simulink model "SGBMDisparityCopy"  (R2021a)
settings: Solver=FixedStepDiscrete  StartTime=0.0  StopTime=simT  FixedStep=1  RelTol=1e-3
PreLoadFcn:
  | DL128 = Simulink.Variant('disparityLevels==128');
  | 
  | DLnot128 = Simulink.Variant('disparityLevels ~= 128');
  | 
  | disparityLevels = 64;
  | 
  | imgRowSize = 480;
  | 
  | imgColSize = 640;
  | 
  | P2 = 200; % Smoothness Penalty Large
  | P1 = 15;  % Smoothness Penalty Small
  | 
  | disparityFactor = 16;
  | 
  | uniquenessRatio = 5;
  | 
  | p = imgColSize - 1;
  | q = imgRowSize * imgColSize -1;
  | r = imgColSize - disparityLevels -1;
  | s = (imgRowSize*(imgColSize-disparityLevels))-1;
  | 
  | simT = 800*525
  | 
  | dtGain = 4;
InitFcn:
  | DL128 = Simulink.Variant('disparityLevels==128');
  | 
  | DLnot128 = Simulink.Variant('disparityLevels ~= 128');
  | 
  | img = imread(get_param('SGBMDisparity/stereoImage','FileName'));
  | 
  | [imgRowSize, imgColSize,chn] = size(img);
  | 
  | P2 = 200; % Smoothness Penalty Large
  | P1 = 15;  % Smoothness Penalty Small
  | 
  | disparityFactor = 16;
  | 
  | uniquenessRatio = str2num(get_param('SGBMDisparity/SGBMHDLAlgorithm/SGBMHDLAlgorithmWorker','UT'));
  | 
  | disparityLevels = str2num(get_param('SGBMDisparity/SGBMHDLAlgorithm/SGBMHDLAlgorithmWorker','DL'));
  | 
  | p = imgColSize - 1;
  | q = imgRowSize * imgColSize -1;
  | r = imgColSize - disparityLevels -1;
  | s = (imgRowSize*(imgColSize-disparityLevels))-1;
  | 
  | if imgRowSize == 720 && imgColSize == 1280
  | simT = 1650*750;
  | elseif imgRowSize == 540 && imgColSize == 960
  | simT = 1050*600;
  | elseif imgRowSize == 480 && imgColSize == 640
  | simT = 800*525;
  | end
  | 
  | if imgRowSize == 720 && imgColSize == 1280
  | dtGain = 2;
  | elseif imgRowSize == 540 && imgColSize == 960
  | dtGain = 2.6;
  | elseif imgRowSize == 480 && imgColSize == 640
  | dtGain = 4;
  | end
undefined symbols (not defined in the file or in its folder): gray
libraries: simulink x331, hdlsllib x113, visionhdlutilities x9, visionhdlio x2, visionsources x1
(part 4 of 6)

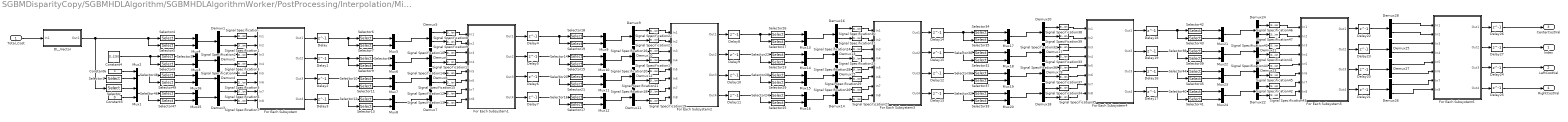
== system SGBMDisparityCopy/SGBMHDLAlgorithm/SGBMHDLAlgorithmWorker/PostProcessing/Interpolation/Minimum_Cost_Index ==
  Total_Cost : Inport
  Constant4 : Constant  Value=[1:128]  OutDataTypeStr=uint8  SampleTime=-1
  Constant5 : Constant  Value=0  OutDataTypeStr=fixdt(1,13,0)  SampleTime=-1
  Constant6 : Constant  Value=0  OutDataTypeStr=fixdt(1,13,0)  SampleTime=-1
  DL_Vector : Subsystem  Variant=on
  Delay{,1..27} (28 alike) : Delay  DelayLength=1
  Demux{1..28} (28 alike) : Demux  Outputs=2
  For Each Subsystem : Subsystem  TreatAsAtomicUnit=on
  For Each Subsystem1 : Subsystem  TreatAsAtomicUnit=on
  For Each Subsystem2 : Subsystem  TreatAsAtomicUnit=on
  For Each Subsystem3 : Subsystem  TreatAsAtomicUnit=on
  For Each Subsystem4 : Subsystem  TreatAsAtomicUnit=on
  For Each Subsystem5 : Subsystem  TreatAsAtomicUnit=on
  For Each Subsystem6 : Subsystem  TreatAsAtomicUnit=on
  Mux{1..26} (26 alike) : Mux  Inputs=2
  Selector : Selector  InputPortWidth=128  IndexOptions=Index vector (dialog)  Indices=[2:128]  OutputSizes=1
  Selector1 : Selector  InputPortWidth=128  IndexOptions=Index vector (dialog)  Indices=[1:127]  OutputSizes=1
  Selector{6,8,10,12} (4 alike) : Selector  InputPortWidth=64  IndexOptions=Index vector (dialog)  Indices=[1:2:64]  OutputSizes=1
  Selector{7,9,11,13} (4 alike) : Selector  InputPortWidth=64  IndexOptions=Index vector (dialog)  Indices=[2:2:64]  OutputSizes=1
  Selector{14,16,18,20} (4 alike) : Selector  InputPortWidth=32  IndexOptions=Index vector (dialog)  Indices=[1:2:32]  OutputSizes=1
  Selector{15,17,19,21} (4 alike) : Selector  InputPortWidth=32  IndexOptions=Index vector (dialog)  Indices=[2:2:32]  OutputSizes=1
  Selector{2,4,46,48} (4 alike) : Selector  InputPortWidth=128  IndexOptions=Index vector (dialog)  Indices=[1:2:128]  OutputSizes=1
  Selector{22,24,26,28} (4 alike) : Selector  InputPortWidth=16  IndexOptions=Index vector (dialog)  Indices=[1:2:16]  OutputSizes=1
  Selector{23,25,27,29} (4 alike) : Selector  InputPortWidth=16  IndexOptions=Index vector (dialog)  Indices=[2:2:16]  OutputSizes=1
  Selector{3,5,47,49} (4 alike) : Selector  InputPortWidth=128  IndexOptions=Index vector (dialog)  Indices=[2:2:128]  OutputSizes=1
  Selector{30,32,34,36} (4 alike) : Selector  InputPortWidth=8  IndexOptions=Index vector (dialog)  Indices=[1:2:8]  OutputSizes=1
  Selector{31,33,35,37} (4 alike) : Selector  InputPortWidth=8  IndexOptions=Index vector (dialog)  Indices=[2:2:8]  OutputSizes=1
  Selector{38,40,42,44} (4 alike) : Selector  InputPortWidth=4  IndexOptions=Index vector (dialog)  Indices=[1:2:4]  OutputSizes=1
  Selector{39,41,43,45} (4 alike) : Selector  InputPortWidth=4  IndexOptions=Index vector (dialog)  Indices=[2:2:4]  OutputSizes=1
  Signal Specification{,1..7} (8 alike) : SignalSpecification  Dimensions=64
  Signal Specification{8..15} (8 alike) : SignalSpecification  Dimensions=32
  Signal Specification{16..23} (8 alike) : SignalSpecification  Dimensions=16
  Signal Specification{24..31} (8 alike) : SignalSpecification  Dimensions=8
  Signal Specification{32..39} (8 alike) : SignalSpecification  Dimensions=4
  Signal Specification{40..47} (8 alike) : SignalSpecification  Dimensions=2
  Index : Outport  VectorParamsAs1DForOutWhenUnconnected=off
  LeftCostVal : Outport  Port=2  VectorParamsAs1DForOutWhenUnconnected=off
  CenterCostVal : Outport  Port=3  VectorParamsAs1DForOutWhenUnconnected=off
  RightCostVal : Outport  Port=4  VectorParamsAs1DForOutWhenUnconnected=off
  wires:
  Demux1/1 -> Signal Specification/1
  Demux1/2 -> Signal Specification1/1
  Demux4/1 -> Signal Specification4/1
  Selector1/1 -> Mux2/2
  Demux2/2 -> Signal Specification3/1
  Demux3/1 -> Signal Specification6/1
  Selector/1 -> Mux1/1
  Demux3/2 -> Signal Specification7/1
  Constant6/1 -> Mux2/1
  Constant5/1 -> Mux1/2
  Demux4/2 -> Signal Specification5/1
  Demux2/1 -> Signal Specification2/1
  Signal Specification/1 -> For Each Subsystem/1(In1)
  Signal Specification1/1 -> For Each Subsystem/2(In2)
  Signal Specification2/1 -> For Each Subsystem/3(In3)
  Signal Specification3/1 -> For Each Subsystem/4(In4)
  Signal Specification4/1 -> For Each Subsystem/5(In5)
  Signal Specification7/1 -> For Each Subsystem/8(In8)
  Signal Specification6/1 -> For Each Subsystem/7(In7)
  Signal Specification5/1 -> For Each Subsystem/6(In6)
  Demux5/1 -> Signal Specification8/1
  For Each Subsystem/1(Out1) -> Delay/1
  Demux6/2 -> Signal Specification11/1
  For Each Subsystem/2(Out2) -> Delay1/1
  Demux5/2 -> Signal Specification9/1
  Demux6/1 -> Signal Specification10/1
  For Each Subsystem/3(Out3) -> Delay2/1
  Demux7/2 -> Signal Specification13/1
  For Each Subsystem/4(Out4) -> Delay3/1
  Demux8/1 -> Signal Specification14/1
  Demux8/2 -> Signal Specification15/1
  Demux7/1 -> Signal Specification12/1
  Signal Specification8/1 -> For Each Subsystem1/1(In1)
  Signal Specification9/1 -> For Each Subsystem1/2(In2)
  Signal Specification10/1 -> For Each Subsystem1/3(In3)
  Signal Specification11/1 -> For Each Subsystem1/4(In4)
  Signal Specification14/1 -> For Each Subsystem1/5(In5)
  Signal Specification15/1 -> For Each Subsystem1/6(In6)
  Signal Specification12/1 -> For Each Subsystem1/7(In7)
  Signal Specification13/1 -> For Each Subsystem1/8(In8)
  For Each Subsystem1/2(Out2) -> Delay5/1
  Signal Specification19/1 -> For Each Subsystem2/8(In8)
  Demux11/2 -> Signal Specification19/1
  Signal Specification18/1 -> For Each Subsystem2/7(In7)
  Signal Specification22/1 -> For Each Subsystem2/1(In1)
  Signal Specification16/1 -> For Each Subsystem2/3(In3)
  For Each Subsystem1/4(Out4) -> Delay7/1
  Signal Specification23/1 -> For Each Subsystem2/2(In2)
  Signal Specification17/1 -> For Each Subsystem2/4(In4)
  Demux10/1 -> Signal Specification16/1
  Demux9/2 -> Signal Specification23/1
  Demux12/1 -> Signal Specification20/1
  Signal Specification20/1 -> For Each Subsystem2/5(In5)
  For Each Subsystem1/1(Out1) -> Delay4/1
  Demux10/2 -> Signal Specification17/1
  Signal Specification21/1 -> For Each Subsystem2/6(In6)
  Demux11/1 -> Signal Specification18/1
  Demux9/1 -> Signal Specification22/1
  For Each Subsystem1/3(Out3) -> Delay6/1
  Demux12/2 -> Signal Specification21/1
  For Each Subsystem2/1(Out1) -> Delay8/1
  Demux14/1 -> Signal Specification26/1
  Demux16/1 -> Signal Specification30/1
  Demux13/2 -> Signal Specification25/1
  Demux15/2 -> Signal Specification29/1
  Demux15/1 -> Signal Specification28/1
  Demux13/1 -> Signal Specification24/1
  Demux16/2 -> Signal Specification31/1
  Demux14/2 -> Signal Specification27/1
  Signal Specification28/1 -> For Each Subsystem3/5(In5)
  Signal Specification26/1 -> For Each Subsystem3/7(In7)
  Signal Specification24/1 -> For Each Subsystem3/3(In3)
  Signal Specification29/1 -> For Each Subsystem3/6(In6)
  For Each Subsystem2/4(Out4) -> Delay11/1
  Signal Specification25/1 -> For Each Subsystem3/4(In4)
  Signal Specification31/1 -> For Each Subsystem3/2(In2)
  For Each Subsystem2/2(Out2) -> Delay9/1
  For Each Subsystem2/3(Out3) -> Delay10/1
  Signal Specification27/1 -> For Each Subsystem3/8(In8)
  Signal Specification30/1 -> For Each Subsystem3/1(In1)
  For Each Subsystem3/1(Out1) -> Delay14/1
  Demux18/1 -> Signal Specification34/1
  Demux20/1 -> Signal Specification38/1
  Demux17/2 -> Signal Specification33/1
  Demux19/2 -> Signal Specification37/1
  Demux19/1 -> Signal Specification36/1
  Demux17/1 -> Signal Specification32/1
  Demux20/2 -> Signal Specification39/1
  Demux18/2 -> Signal Specification35/1
  Signal Specification36/1 -> For Each Subsystem4/5(In5)
  Signal Specification34/1 -> For Each Subsystem4/7(In7)
  Signal Specification32/1 -> For Each Subsystem4/3(In3)
  Signal Specification37/1 -> For Each Subsystem4/6(In6)
  For Each Subsystem3/4(Out4) -> Delay13/1
  Signal Specification33/1 -> For Each Subsystem4/4(In4)
  Signal Specification39/1 -> For Each Subsystem4/2(In2)
  For Each Subsystem3/2(Out2) -> Delay15/1
  For Each Subsystem3/3(Out3) -> Delay12/1
  Signal Specification35/1 -> For Each Subsystem4/8(In8)
  Signal Specification38/1 -> For Each Subsystem4/1(In1)
  For Each Subsystem4/1(Out1) -> Delay18/1
  For Each Subsystem4/4(Out4) -> Delay17/1
  For Each Subsystem4/2(Out2) -> Delay19/1
  For Each Subsystem4/3(Out3) -> Delay16/1
  Constant4/1 -> Selector3/1, Selector2/1
  Selector2/1 -> Mux3/1
  Selector3/1 -> Mux3/2
  Mux3/1 -> Demux2/1
  Selector4/1 -> Mux4/1
  Selector5/1 -> Mux4/2
  Mux4/1 -> Demux1/1
  Demux24/1 -> Signal Specification46/1
  Demux24/2 -> Signal Specification47/1
  Demux22/2 -> Signal Specification43/1
  Demux21/2 -> Signal Specification41/1
  Demux23/2 -> Signal Specification45/1
  Demux23/1 -> Signal Specification44/1
  Demux21/1 -> Signal Specification40/1
  Demux22/1 -> Signal Specification42/1
  For Each Subsystem5/2(Out2) -> Delay23/1
  For Each Subsystem5/3(Out3) -> Delay20/1
  For Each Subsystem5/4(Out4) -> Delay21/1
  For Each Subsystem5/1(Out1) -> Delay22/1
  Selector6/1 -> Mux5/1
  Selector7/1 -> Mux5/2
  Delay/1 -> Selector7/1, Selector6/1
  Mux5/1 -> Demux5/1
  Selector8/1 -> Mux6/1
  Selector9/1 -> Mux6/2
  Delay1/1 -> Selector8/1, Selector9/1
  Mux6/1 -> Demux6/1
  Mux7/1 -> Demux8/1
  Selector11/1 -> Mux7/2
  Delay2/1 -> Selector11/1, Selector10/1
  Selector10/1 -> Mux7/1
  Mux8/1 -> Demux7/1
  Selector13/1 -> Mux8/2
  Delay3/1 -> Selector12/1, Selector13/1
  Selector12/1 -> Mux8/1
  Selector20/1 -> Mux11/1
  Selector21/1 -> Mux11/2
  Delay5/1 -> Selector15/1, Selector14/1
  Mux10/1 -> Demux10/1
  Delay6/1 -> Selector20/1, Selector21/1
  Selector17/1 -> Mux12/2
  Mux11/1 -> Demux12/1
  Selector16/1 -> Mux12/1
  Selector15/1 -> Mux10/2
  Mux9/1 -> Demux9/1
  Selector19/1 -> Mux9/2
  Delay4/1 -> Selector19/1, Selector18/1
  Selector18/1 -> Mux9/1
  Selector14/1 -> Mux10/1
  Mux12/1 -> Demux11/1
  Delay7/1 -> Selector17/1, Selector16/1
  Selector28/1 -> Mux15/1
  Selector29/1 -> Mux15/2
  Delay9/1 -> Selector23/1, Selector22/1
  Mux14/1 -> Demux13/1
  Delay10/1 -> Selector29/1, Selector28/1
  Selector25/1 -> Mux16/2
  Mux15/1 -> Demux15/1
  Selector24/1 -> Mux16/1
  Selector23/1 -> Mux14/2
  Mux13/1 -> Demux16/1
  Selector27/1 -> Mux13/2
  Delay8/1 -> Selector27/1, Selector26/1
  Selector26/1 -> Mux13/1
  Selector22/1 -> Mux14/1
  Mux16/1 -> Demux14/1
  Delay11/1 -> Selector25/1, Selector24/1
  Selector36/1 -> Mux19/1
  Selector37/1 -> Mux19/2
  Delay15/1 -> Selector31/1, Selector30/1
  Mux18/1 -> Demux17/1
  Delay12/1 -> Selector37/1, Selector36/1
  Selector33/1 -> Mux20/2
  Mux19/1 -> Demux19/1
  Selector32/1 -> Mux20/1
  Selector31/1 -> Mux18/2
  Mux17/1 -> Demux20/1
  Selector35/1 -> Mux17/2
  Delay14/1 -> Selector35/1, Selector34/1
  Selector34/1 -> Mux17/1
  Selector30/1 -> Mux18/1
  Mux20/1 -> Demux18/1
  Delay13/1 -> Selector33/1, Selector32/1
  Selector44/1 -> Mux23/1
  Selector45/1 -> Mux23/2
  Delay19/1 -> Selector38/1, Selector39/1
  Mux22/1 -> Demux21/1
  Delay16/1 -> Selector45/1, Selector44/1
  Selector41/1 -> Mux24/2
  Mux23/1 -> Demux23/1
  Selector40/1 -> Mux24/1
  Selector39/1 -> Mux22/2
  Mux21/1 -> Demux24/1
  Selector43/1 -> Mux21/2
  Delay18/1 -> Selector43/1, Selector42/1
  Selector42/1 -> Mux21/1
  Selector38/1 -> Mux22/1
  Mux24/1 -> Demux22/1
  Delay17/1 -> Selector41/1, Selector40/1
  Mux2/1 -> Selector49/1, Selector48/1
  Mux25/1 -> Demux3/1
  Selector47/1 -> Mux25/2
  Selector48/1 -> Mux26/1
  Mux1/1 -> Selector47/1, Selector46/1
  Selector49/1 -> Mux26/2
  Mux26/1 -> Demux4/1
  Selector46/1 -> Mux25/1
  DL_Vector/1(Out1) -> Selector1/1, Selector/1, Selector5/1, Selector4/1
  Signal Specification42/1 -> For Each Subsystem5/7(In7)
  Signal Specification41/1 -> For Each Subsystem5/4(In4)
  Signal Specification40/1 -> For Each Subsystem5/3(In3)
  Signal Specification45/1 -> For Each Subsystem5/6(In6)
  Signal Specification46/1 -> For Each Subsystem5/1(In1)
  Signal Specification43/1 -> For Each Subsystem5/8(In8)
  Signal Specification44/1 -> For Each Subsystem5/5(In5)
  Signal Specification47/1 -> For Each Subsystem5/2(In2)
  For Each Subsystem6/2(Out2) -> Delay27/1
  For Each Subsystem6/3(Out3) -> Delay24/1
  Demux26/2 -> For Each Subsystem6/8(In8)
  Demux28/1 -> For Each Subsystem6/1(In1)
  Demux27/2 -> For Each Subsystem6/6(In6)
  Demux25/2 -> For Each Subsystem6/4(In4)
  For Each Subsystem6/4(Out4) -> Delay25/1
  Delay21/1 -> Demux26/1
  Delay20/1 -> Demux27/1
  Demux28/2 -> For Each Subsystem6/2(In2)
  For Each Subsystem6/1(Out1) -> Delay26/1
  Demux27/1 -> For Each Subsystem6/5(In5)
  Delay23/1 -> Demux25/1
  Demux25/1 -> For Each Subsystem6/3(In3)
  Demux26/1 -> For Each Subsystem6/7(In7)
  Delay22/1 -> Demux28/1
  Delay26/1 -> CenterCostVal/1
  Delay27/1 -> Index/1
  Delay24/1 -> LeftCostVal/1
  Delay25/1 -> RightCostVal/1
  Total_Cost/1 -> DL_Vector/1(In1)

== system SGBMDisparityCopy/SGBMHDLAlgorithm/SGBMHDLAlgorithmWorker/PostProcessing/UniquenessFcn/For Each Subsystem ==
  total_cost : Inport  Partition=on  PartitionDimension=1  PartitionWidth=1  PartitionOffset=0
  total_cost1 : Inport  Port=2
  min_index_val : Inport  Port=3
  Delay : Delay  DelayLength=1
  For Each : ForEach  DisableCoverage=on
  Product : Product  RndMeth=Simplest
  Relational Operator1 : RelationalOperator  Operator=<  OutDataTypeStr=boolean  RndMeth=Nearest
  Out1 : Outport  ConcatenationDimension=1  VectorParamsAs1DForOutWhenUnconnected=off
  wires:
  total_cost/1 -> Product/1
  total_cost1/1 -> Product/2
  Product/1 -> Delay/1
  Delay/1 -> Relational Operator1/1
  min_index_val/1 -> Relational Operator1/2
  Relational Operator1/1 -> Out1/1

== system SGBMDisparityCopy/SGBMHDLAlgorithm/SGBMHDLAlgorithmWorker/PostProcessing/UniquenessFcn/For Each Subsystem1 ==
  min_Index : Inport
  Index : Inport  Port=2  Partition=on  PartitionDimension=1  PartitionWidth=1  PartitionOffset=0
  Abs1 : Abs  RndMeth=Simplest  SaturateOnIntegerOverflow=on
  Add2 : Sum  Inputs=+-
  Constant63 : Constant  OutDataTypeStr=uint8  SampleTime=-1
  Delay133 : Delay  DelayLength=1
  Delay37 : Delay  DelayLength=1
  For Each : ForEach  DisableCoverage=on
  Relational Operator2 : RelationalOperator  Operator=>  OutDataTypeStr=boolean  RndMeth=Nearest
  Out1 : Outport  ConcatenationDimension=1  VectorParamsAs1DForOutWhenUnconnected=off
  wires:
  Add2/1 -> Delay133/1
  Constant63/1 -> Relational Operator2/2
  Abs1/1 -> Delay37/1
  Delay37/1 -> Relational Operator2/1
  Delay133/1 -> Abs1/1
  min_Index/1 -> Add2/1
  Index/1 -> Add2/2
  Relational Operator2/1 -> Out1/1

== system SGBMDisparityCopy/SGBMHDLAlgorithm/SGBMHDLAlgorithmWorker/DirectionalCost/LeftToRight/lrSubsystem/For Each Subsystem ==
  In1 : Inport  Partition=on  PartitionDimension=1  PartitionWidth=1  PartitionOffset=0
  Constant2 : Constant  Value=0  OutDataTypeStr=boolean  SampleTime=-1
  For Each : ForEach  DisableCoverage=on
  Terminator : Terminator
  Out1 : Outport  ConcatenationDimension=1  VectorParamsAs1DForOutWhenUnconnected=off
  wires:
  Constant2/1 -> Out1/1
  In1/1 -> Terminator/1

== system SGBMDisparityCopy/SGBMHDLAlgorithm/SGBMHDLAlgorithmWorker/DirectionalCost/LeftToRight/lrSubsystem/d+1 ==
  prevCost_d : Inport
  Constant : Constant  Value=255  OutDataTypeStr=fixdt(1,10,0)  SampleTime=-1
  Selector : Selector  InputPortWidth=disparityLevels  IndexOptions=Index vector (dialog)  Indices=[2:disparityLevels]  OutputSizes=1
  Vector Concatenate : Concatenate
  prevCost_d+1 : Outport  VectorParamsAs1DForOutWhenUnconnected=off
  wires:
  prevCost_d/1 -> Selector/1
  Vector Concatenate/1 -> prevCost_d+1/1
  Selector/1 -> Vector Concatenate/1
  Constant/1 -> Vector Concatenate/2

== system SGBMDisparityCopy/SGBMHDLAlgorithm/SGBMHDLAlgorithmWorker/DirectionalCost/LeftToRight/lrSubsystem/d-1 ==
  prevCost_d : Inport
  Constant : Constant  Value=255  OutDataTypeStr=fixdt(1,10,0)  SampleTime=-1
  Selector : Selector  InputPortWidth=disparityLevels  IndexOptions=Index vector (dialog)  Indices=[1:disparityLevels-1]  OutputSizes=1
  Vector Concatenate : Concatenate
  prevCost_d-1 : Outport  VectorParamsAs1DForOutWhenUnconnected=off
  wires:
  prevCost_d/1 -> Selector/1
  Vector Concatenate/1 -> prevCost_d-1/1
  Selector/1 -> Vector Concatenate/2
  Constant/1 -> Vector Concatenate/1

== system SGBMDisparityCopy/SGBMHDLAlgorithm/SGBMHDLAlgorithmWorker/DirectionalCost/LeftToRight/lrSubsystem/minCostPath ==
  matchingCost : Inport  Partition=on  PartitionDimension=1  PartitionWidth=1  PartitionOffset=0
  prevCost_d : Inport  Port=2  Partition=on  PartitionDimension=1  PartitionWidth=1  PartitionOffset=0
  prevCost_d-1 : Inport  Port=3  Partition=on  PartitionDimension=1  PartitionWidth=1  PartitionOffset=0
  prevCost_d+1 : Inport  Port=4  Partition=on  PartitionDimension=1  PartitionWidth=1  PartitionOffset=0
  minPrevCost : Inport  Port=5
  Constant : Constant  Value=P1  OutDataTypeStr=fixdt(0,5,0)  SampleTime=-1
  Constant1 : Constant  Value=P2  OutDataTypeStr=uint8  SampleTime=-1
  For Each : ForEach  DisableCoverage=on
  Min : MinMax  Inputs=4
  Sum : Sum  Inputs=|++  OutDataTypeStr=fixdt(0,13,0)  SaturateOnIntegerOverflow=on
  Sum1 : Sum  Inputs=++|  OutDataTypeStr=fixdt(0,13,0)  SaturateOnIntegerOverflow=on
  Sum2 : Sum  Inputs=++|  OutDataTypeStr=int16  SaturateOnIntegerOverflow=on
  Sum3 : Sum  OutDataTypeStr=fixdt(1,17,0)  SaturateOnIntegerOverflow=on
  Sum4 : Sum  Inputs=+-  OutDataTypeStr=fixdt(1,10,0)  SaturateOnIntegerOverflow=on
  currCost : Outport  ConcatenationDimension=1  VectorParamsAs1DForOutWhenUnconnected=off
  wires:
  Sum1/1 -> Min/3
  Sum2/1 -> Min/4
  minPrevCost/1 -> Sum4/2, Sum2/2
  Sum/1 -> Min/2
  Constant1/1 -> Sum2/1
  prevCost_d/1 -> Min/1
  prevCost_d-1/1 -> Sum/1
  Min/1 -> Sum3/2
  prevCost_d+1/1 -> Sum1/2
  Constant/1 -> Sum1/1, Sum/2
  matchingCost/1 -> Sum3/1
  Sum3/1 -> Sum4/1
  Sum4/1 -> currCost/1

== system SGBMDisparityCopy/SGBMHDLAlgorithm/SGBMHDLAlgorithmWorker/DirectionalCost/RightToLeft/rlSubsystem/For Each Subsystem ==
  In1 : Inport  Partition=on  PartitionDimension=1  PartitionWidth=1  PartitionOffset=0
  Constant2 : Constant  Value=0  OutDataTypeStr=boolean  SampleTime=-1
  For Each : ForEach  DisableCoverage=on
  Terminator : Terminator
  Out1 : Outport  ConcatenationDimension=1  VectorParamsAs1DForOutWhenUnconnected=off
  wires:
  Constant2/1 -> Out1/1
  In1/1 -> Terminator/1

== system SGBMDisparityCopy/SGBMHDLAlgorithm/SGBMHDLAlgorithmWorker/DirectionalCost/RightToLeft/rlSubsystem/d+1 ==
  prev_cost_d : Inport
  Constant : Constant  Value=255  OutDataTypeStr=fixdt(1,10,0)  SampleTime=-1
  Selector : Selector  InputPortWidth=disparityLevels  IndexOptions=Index vector (dialog)  Indices=[2:disparityLevels]  OutputSizes=1
  Vector Concatenate : Concatenate
  prev_cost_d+1 : Outport  VectorParamsAs1DForOutWhenUnconnected=off
  wires:
  prev_cost_d/1 -> Selector/1
  Vector Concatenate/1 -> prev_cost_d+1/1
  Selector/1 -> Vector Concatenate/1
  Constant/1 -> Vector Concatenate/2

== system SGBMDisparityCopy/SGBMHDLAlgorithm/SGBMHDLAlgorithmWorker/DirectionalCost/RightToLeft/rlSubsystem/d-1 ==
  prev_cost_d : Inport
  Constant : Constant  Value=255  OutDataTypeStr=fixdt(1,10,0)  SampleTime=-1
  Selector : Selector  InputPortWidth=disparityLevels  IndexOptions=Index vector (dialog)  Indices=[1:disparityLevels-1]  OutputSizes=1
  Vector Concatenate : Concatenate
  prev_cost_d-1 : Outport  VectorParamsAs1DForOutWhenUnconnected=off
  wires:
  prev_cost_d/1 -> Selector/1
  Vector Concatenate/1 -> prev_cost_d-1/1
  Selector/1 -> Vector Concatenate/2
  Constant/1 -> Vector Concatenate/1

== system SGBMDisparityCopy/SGBMHDLAlgorithm/SGBMHDLAlgorithmWorker/DirectionalCost/RightToLeft/rlSubsystem/minCostPath ==
  Matching_Cost : Inport  Partition=on  PartitionDimension=1  PartitionWidth=1  PartitionOffset=0
  prev_cost_d : Inport  Port=2  Partition=on  PartitionDimension=1  PartitionWidth=1  PartitionOffset=0
  prev_cost_d-1 : Inport  Port=3  Partition=on  PartitionDimension=1  PartitionWidth=1  PartitionOffset=0
  prev_cost_d+1 : Inport  Port=4  Partition=on  PartitionDimension=1  PartitionWidth=1  PartitionOffset=0
  min_prev_cost : Inport  Port=5
  Constant : Constant  Value=P1  OutDataTypeStr=fixdt(0,5,0)  SampleTime=-1
  Constant1 : Constant  Value=P2  OutDataTypeStr=uint8  SampleTime=-1
  For Each : ForEach  DisableCoverage=on
  Min : MinMax  Inputs=4
  Sum : Sum  Inputs=|++  OutDataTypeStr=fixdt(0,13,0)  SaturateOnIntegerOverflow=on
  Sum1 : Sum  Inputs=++|  OutDataTypeStr=fixdt(0,13,0)  SaturateOnIntegerOverflow=on
  Sum2 : Sum  Inputs=++|  OutDataTypeStr=int16  SaturateOnIntegerOverflow=on
  Sum3 : Sum  OutDataTypeStr=fixdt(1,17,0)  SaturateOnIntegerOverflow=on
  Sum4 : Sum  Inputs=+-  OutDataTypeStr=fixdt(1,10,0)  SaturateOnIntegerOverflow=on
  curr_cost : Outport  ConcatenationDimension=1  VectorParamsAs1DForOutWhenUnconnected=off
  wires:
  Sum1/1 -> Min/3
  Sum2/1 -> Min/4
  Sum3/1 -> Sum4/1
  min_prev_cost/1 -> Sum4/2, Sum2/2
  Sum/1 -> Min/2
  Constant1/1 -> Sum2/1
  prev_cost_d/1 -> Min/1
  prev_cost_d-1/1 -> Sum/1
  Min/1 -> Sum3/2
  prev_cost_d+1/1 -> Sum1/2
  Constant/1 -> Sum1/1, Sum/2
  Matching_Cost/1 -> Sum3/1
  Sum4/1 -> curr_cost/1

== system SGBMDisparityCopy/SGBMHDLAlgorithm/SGBMHDLAlgorithmWorker/DirectionalCost/TopLeftToBottomRight/tlbrSubsystem/For Each Subsystem ==
  In1 : Inport  Partition=on  PartitionDimension=1  PartitionWidth=1  PartitionOffset=0
  Constant2 : Constant  Value=0  OutDataTypeStr=boolean  SampleTime=-1
  For Each : ForEach  DisableCoverage=on
  Terminator : Terminator
  Out1 : Outport  ConcatenationDimension=1  VectorParamsAs1DForOutWhenUnconnected=off
  wires:
  Constant2/1 -> Out1/1
  In1/1 -> Terminator/1

== system SGBMDisparityCopy/SGBMHDLAlgorithm/SGBMHDLAlgorithmWorker/DirectionalCost/TopLeftToBottomRight/tlbrSubsystem/d+2 ==
  prev_cost_d : Inport
  Constant : Constant  Value=255  OutDataTypeStr=fixdt(1,10,0)  SampleTime=-1
  Selector : Selector  InputPortWidth=disparityLevels  IndexOptions=Index vector (dialog)  Indices=[2:disparityLevels]  OutputSizes=1
  Vector Concatenate : Concatenate
  prev_cost_d+1 : Outport  VectorParamsAs1DForOutWhenUnconnected=off
  wires:
  prev_cost_d/1 -> Selector/1
  Vector Concatenate/1 -> prev_cost_d+1/1
  Selector/1 -> Vector Concatenate/1
  Constant/1 -> Vector Concatenate/2

== system SGBMDisparityCopy/SGBMHDLAlgorithm/SGBMHDLAlgorithmWorker/DirectionalCost/TopLeftToBottomRight/tlbrSubsystem/d-2 ==
  prev_cost_d : Inport
  Constant : Constant  Value=255  OutDataTypeStr=fixdt(1,10,0)  SampleTime=-1
  Selector : Selector  InputPortWidth=disparityLevels  IndexOptions=Index vector (dialog)  Indices=[1:disparityLevels-1]  OutputSizes=1
  Vector Concatenate : Concatenate
  prev_cost_d-1 : Outport  VectorParamsAs1DForOutWhenUnconnected=off
  wires:
  prev_cost_d/1 -> Selector/1
  Vector Concatenate/1 -> prev_cost_d-1/1
  Selector/1 -> Vector Concatenate/2
  Constant/1 -> Vector Concatenate/1

== system SGBMDisparityCopy/SGBMHDLAlgorithm/SGBMHDLAlgorithmWorker/DirectionalCost/TopLeftToBottomRight/tlbrSubsystem/minCostPath ==
  Matching_Cost : Inport  Partition=on  PartitionDimension=1  PartitionWidth=1  PartitionOffset=0
  prev_cost_d : Inport  Port=2  Partition=on  PartitionDimension=1  PartitionWidth=1  PartitionOffset=0
  prev_cost_d-1 : Inport  Port=3  Partition=on  PartitionDimension=1  PartitionWidth=1  PartitionOffset=0
  prev_cost_d+1 : Inport  Port=4  Partition=on  PartitionDimension=1  PartitionWidth=1  PartitionOffset=0
  min_prev_cost : Inport  Port=5
  Constant : Constant  Value=P1  OutDataTypeStr=fixdt(0,5,0)  SampleTime=-1
  Constant1 : Constant  Value=P2  OutDataTypeStr=uint8  SampleTime=-1
  For Each : ForEach  DisableCoverage=on
  Min : MinMax  Inputs=4
  Sum : Sum  Inputs=|++  OutDataTypeStr=fixdt(0,13,0)  SaturateOnIntegerOverflow=on
  Sum1 : Sum  Inputs=++|  OutDataTypeStr=fixdt(0,13,0)  SaturateOnIntegerOverflow=on
  Sum2 : Sum  Inputs=++|  OutDataTypeStr=int16  SaturateOnIntegerOverflow=on
  Sum3 : Sum  OutDataTypeStr=fixdt(1,17,0)  SaturateOnIntegerOverflow=on
  Sum4 : Sum  Inputs=+-  OutDataTypeStr=fixdt(1,10,0)  SaturateOnIntegerOverflow=on
  curr_cost : Outport  ConcatenationDimension=1  VectorParamsAs1DForOutWhenUnconnected=off
  wires:
  Sum1/1 -> Min/3
  Sum2/1 -> Min/4
  Sum3/1 -> Sum4/1
  min_prev_cost/1 -> Sum4/2, Sum2/2
  Sum/1 -> Min/2
  Constant1/1 -> Sum2/1
  prev_cost_d/1 -> Min/1
  prev_cost_d-1/1 -> Sum/1
  Min/1 -> Sum3/2
  prev_cost_d+1/1 -> Sum1/2
  Constant/1 -> Sum1/1, Sum/2
  Matching_Cost/1 -> Sum3/1
  Sum4/1 -> curr_cost/1

== system SGBMDisparityCopy/SGBMHDLAlgorithm/SGBMHDLAlgorithmWorker/DirectionalCost/TopRightToBottomLeft/trblSubsystem/For Each Subsystem ==
  In1 : Inport  Partition=on  PartitionDimension=1  PartitionWidth=1  PartitionOffset=0
  Constant2 : Constant  Value=0  OutDataTypeStr=boolean  SampleTime=-1
  For Each : ForEach  DisableCoverage=on
  Terminator : Terminator
  Out1 : Outport  ConcatenationDimension=1  VectorParamsAs1DForOutWhenUnconnected=off
  wires:
  Constant2/1 -> Out1/1
  In1/1 -> Terminator/1

== system SGBMDisparityCopy/SGBMHDLAlgorithm/SGBMHDLAlgorithmWorker/DirectionalCost/TopRightToBottomLeft/trblSubsystem/d+2 ==
  prev_cost_d : Inport
  Constant : Constant  Value=255  OutDataTypeStr=fixdt(1,10,0)  SampleTime=-1
  Selector : Selector  InputPortWidth=disparityLevels  IndexOptions=Index vector (dialog)  Indices=[2:disparityLevels]  OutputSizes=1
  Vector Concatenate : Concatenate
  prev_cost_d+1 : Outport  VectorParamsAs1DForOutWhenUnconnected=off
  wires:
  prev_cost_d/1 -> Selector/1
  Vector Concatenate/1 -> prev_cost_d+1/1
  Selector/1 -> Vector Concatenate/1
  Constant/1 -> Vector Concatenate/2

== system SGBMDisparityCopy/SGBMHDLAlgorithm/SGBMHDLAlgorithmWorker/DirectionalCost/TopRightToBottomLeft/trblSubsystem/d-2 ==
  prev_cost_d : Inport
  Constant : Constant  Value=255  OutDataTypeStr=fixdt(1,10,0)  SampleTime=-1
  Selector : Selector  InputPortWidth=disparityLevels  IndexOptions=Index vector (dialog)  Indices=[1:disparityLevels-1]  OutputSizes=1
  Vector Concatenate : Concatenate
  prev_cost_d-1 : Outport  VectorParamsAs1DForOutWhenUnconnected=off
  wires:
  prev_cost_d/1 -> Selector/1
  Vector Concatenate/1 -> prev_cost_d-1/1
  Selector/1 -> Vector Concatenate/2
  Constant/1 -> Vector Concatenate/1

== system SGBMDisparityCopy/SGBMHDLAlgorithm/SGBMHDLAlgorithmWorker/DirectionalCost/TopRightToBottomLeft/trblSubsystem/minCostPath ==
  Matching_Cost : Inport  Partition=on  PartitionDimension=1  PartitionWidth=1  PartitionOffset=0
  prev_cost_d : Inport  Port=2  Partition=on  PartitionDimension=1  PartitionWidth=1  PartitionOffset=0
  prev_cost_d-1 : Inport  Port=3  Partition=on  PartitionDimension=1  PartitionWidth=1  PartitionOffset=0
  prev_cost_d+1 : Inport  Port=4  Partition=on  PartitionDimension=1  PartitionWidth=1  PartitionOffset=0
  min_prev_cost : Inport  Port=5
  Constant : Constant  Value=P1  OutDataTypeStr=fixdt(0,5,0)  SampleTime=-1
  Constant1 : Constant  Value=P2  OutDataTypeStr=uint8  SampleTime=-1
  For Each : ForEach  DisableCoverage=on
  Min : MinMax  Inputs=4
  Sum : Sum  Inputs=|++  OutDataTypeStr=fixdt(0,13,0)  SaturateOnIntegerOverflow=on
  Sum1 : Sum  Inputs=++|  OutDataTypeStr=fixdt(0,13,0)  SaturateOnIntegerOverflow=on
  Sum2 : Sum  Inputs=++|  OutDataTypeStr=int16  SaturateOnIntegerOverflow=on
  Sum3 : Sum  OutDataTypeStr=fixdt(1,17,0)  SaturateOnIntegerOverflow=on
  Sum4 : Sum  Inputs=+-  OutDataTypeStr=fixdt(1,10,0)  SaturateOnIntegerOverflow=on
  curr_cost : Outport  ConcatenationDimension=1  VectorParamsAs1DForOutWhenUnconnected=off
  wires:
  Sum1/1 -> Min/3
  Sum2/1 -> Min/4
  min_prev_cost/1 -> Sum4/2, Sum2/2
  Sum/1 -> Min/2
  Constant1/1 -> Sum2/1
  prev_cost_d/1 -> Min/1
  prev_cost_d-1/1 -> Sum/1
  Min/1 -> Sum3/2
  prev_cost_d+1/1 -> Sum1/2
  Constant/1 -> Sum1/1, Sum/2
  Matching_Cost/1 -> Sum3/1
  Sum3/1 -> Sum4/1
  Sum4/1 -> curr_cost/1

== system SGBMDisparityCopy/SGBMHDLAlgorithm/SGBMHDLAlgorithmWorker/DirectionalCost/TopToBottom/tbSubsystem/For Each Subsystem ==
  In1 : Inport  Partition=on  PartitionDimension=1  PartitionWidth=1  PartitionOffset=0
  Constant2 : Constant  Value=0  OutDataTypeStr=boolean  SampleTime=-1
  For Each : ForEach  DisableCoverage=on
  Terminator : Terminator
  Out1 : Outport  ConcatenationDimension=1  VectorParamsAs1DForOutWhenUnconnected=off
  wires:
  Constant2/1 -> Out1/1
  In1/1 -> Terminator/1

== system SGBMDisparityCopy/SGBMHDLAlgorithm/SGBMHDLAlgorithmWorker/DirectionalCost/TopToBottom/tbSubsystem/d+1 ==
  prev_cost_d : Inport
  Constant : Constant  Value=255  OutDataTypeStr=fixdt(1,10,0)  SampleTime=-1
  Selector : Selector  InputPortWidth=disparityLevels  IndexOptions=Index vector (dialog)  Indices=[2:disparityLevels]  OutputSizes=1
  Vector Concatenate : Concatenate
  prev_cost_d+1 : Outport  VectorParamsAs1DForOutWhenUnconnected=off
  wires:
  prev_cost_d/1 -> Selector/1
  Vector Concatenate/1 -> prev_cost_d+1/1
  Selector/1 -> Vector Concatenate/1
  Constant/1 -> Vector Concatenate/2

== system SGBMDisparityCopy/SGBMHDLAlgorithm/SGBMHDLAlgorithmWorker/DirectionalCost/TopToBottom/tbSubsystem/d-1 ==
  prev_cost_d : Inport
  Constant : Constant  Value=255  OutDataTypeStr=fixdt(1,10,0)  SampleTime=-1
  Selector : Selector  InputPortWidth=disparityLevels  IndexOptions=Index vector (dialog)  Indices=[1:disparityLevels-1]  OutputSizes=1
  Vector Concatenate : Concatenate
  prev_cost_d-1 : Outport  VectorParamsAs1DForOutWhenUnconnected=off
  wires:
  prev_cost_d/1 -> Selector/1
  Vector Concatenate/1 -> prev_cost_d-1/1
  Selector/1 -> Vector Concatenate/2
  Constant/1 -> Vector Concatenate/1

== system SGBMDisparityCopy/SGBMHDLAlgorithm/SGBMHDLAlgorithmWorker/DirectionalCost/TopToBottom/tbSubsystem/minCostPath ==
  Matching_Cost : Inport  Partition=on  PartitionDimension=1  PartitionWidth=1  PartitionOffset=0
  prev_cost_d : Inport  Port=2  Partition=on  PartitionDimension=1  PartitionWidth=1  PartitionOffset=0
  prev_cost_d-1 : Inport  Port=3  Partition=on  PartitionDimension=1  PartitionWidth=1  PartitionOffset=0
  prev_cost_d+1 : Inport  Port=4  Partition=on  PartitionDimension=1  PartitionWidth=1  PartitionOffset=0
  min_prev_cost : Inport  Port=5
  Constant : Constant  Value=P1  OutDataTypeStr=fixdt(0,5,0)  SampleTime=-1
  Constant1 : Constant  Value=P2  OutDataTypeStr=uint8  SampleTime=-1
  For Each : ForEach  DisableCoverage=on
  Min : MinMax  Inputs=4
  Sum : Sum  Inputs=|++  OutDataTypeStr=fixdt(0,13,0)  SaturateOnIntegerOverflow=on
  Sum1 : Sum  Inputs=++|  OutDataTypeStr=fixdt(0,13,0)  SaturateOnIntegerOverflow=on
  Sum2 : Sum  Inputs=++|  OutDataTypeStr=int16  SaturateOnIntegerOverflow=on
  Sum3 : Sum  OutDataTypeStr=fixdt(1,17,0)  SaturateOnIntegerOverflow=on
  Sum4 : Sum  Inputs=+-  OutDataTypeStr=fixdt(1,10,0)  SaturateOnIntegerOverflow=on
  curr_cost : Outport  ConcatenationDimension=1  VectorParamsAs1DForOutWhenUnconnected=off
  wires:
  Sum1/1 -> Min/3
  Sum2/1 -> Min/4
  Sum3/1 -> Sum4/1
  min_prev_cost/1 -> Sum4/2, Sum2/2
  Sum/1 -> Min/2
  Constant1/1 -> Sum2/1
  prev_cost_d/1 -> Min/1
  prev_cost_d-1/1 -> Sum/1
  Min/1 -> Sum3/2
  prev_cost_d+1/1 -> Sum1/2
  Constant/1 -> Sum1/1, Sum/2
  Matching_Cost/1 -> Sum3/1
  Sum4/1 -> curr_cost/1

== system SGBMDisparityCopy/SGBMHDLAlgorithm/SGBMHDLAlgorithmWorker/MatchingCost/CensusTransform/ctLogic/For Each Subsystem ==
  In1 : Inport  Partition=on  PartitionDimension=1  PartitionWidth=1  PartitionOffset=0
  In2 : Inport  Port=2  Partition=on  PartitionDimension=1  PartitionWidth=1  PartitionOffset=0
  For Each : ForEach  DisableCoverage=on
  Relational Operator : RelationalOperator  OutDataTypeStr=boolean  RndMeth=Nearest
  Out1 : Outport  ConcatenationDimension=1  VectorParamsAs1DForOutWhenUnconnected=off
  wires:
  In1/1 -> Relational Operator/1
  In2/1 -> Relational Operator/2
  Relational Operator/1 -> Out1/1

== system SGBMDisparityCopy/SGBMHDLAlgorithm/SGBMHDLAlgorithmWorker/MatchingCost/CensusTransform/ctLogic/For Each Subsystem1 ==
  In1 : Inport  Partition=on  PartitionDimension=1  PartitionWidth=1  PartitionOffset=0
  In2 : Inport  Port=2  Partition=on  PartitionDimension=1  PartitionWidth=1  PartitionOffset=0
  For Each : ForEach  DisableCoverage=on
  Relational Operator : RelationalOperator  OutDataTypeStr=boolean  RndMeth=Nearest
  Out1 : Outport  ConcatenationDimension=1  VectorParamsAs1DForOutWhenUnconnected=off
  wires:
  In1/1 -> Relational Operator/1
  In2/1 -> Relational Operator/2
  Relational Operator/1 -> Out1/1

== system SGBMDisparityCopy/SGBMHDLAlgorithm/SGBMHDLAlgorithmWorker/MatchingCost/CensusTransform/ctLogic/For Each Subsystem2 ==
  In1 : Inport  Partition=on  PartitionDimension=1  PartitionWidth=1  PartitionOffset=0
  In2 : Inport  Port=2  Partition=on  PartitionDimension=1  PartitionWidth=1  PartitionOffset=0
  For Each : ForEach  DisableCoverage=on
  Relational Operator : RelationalOperator  OutDataTypeStr=boolean  RndMeth=Nearest
  Out1 : Outport  ConcatenationDimension=1  VectorParamsAs1DForOutWhenUnconnected=off
  wires:
  In1/1 -> Relational Operator/1
  In2/1 -> Relational Operator/2
  Relational Operator/1 -> Out1/1

== system SGBMDisparityCopy/SGBMHDLAlgorithm/SGBMHDLAlgorithmWorker/MatchingCost/CensusTransform/ctLogic/For Each Subsystem3 ==
  In1 : Inport  Partition=on  PartitionDimension=1  PartitionWidth=1  PartitionOffset=0
  In2 : Inport  Port=2  Partition=on  PartitionDimension=1  PartitionWidth=1  PartitionOffset=0
  For Each : ForEach  DisableCoverage=on
  Relational Operator : RelationalOperator  OutDataTypeStr=boolean  RndMeth=Nearest
  Out1 : Outport  ConcatenationDimension=1  VectorParamsAs1DForOutWhenUnconnected=off
  wires:
  In1/1 -> Relational Operator/1
  In2/1 -> Relational Operator/2
  Relational Operator/1 -> Out1/1

== system SGBMDisparityCopy/SGBMHDLAlgorithm/SGBMHDLAlgorithmWorker/MatchingCost/CensusTransform/dataAligner/pixelBusGenerator ==
  validIn : Inport
  Horizontal : hdlsllib/Sources/HDL Counter  CountType=Count limited  CountInit=0  CountStep=1  CountMax=hEnd  CountFromType=Initial value  CountFrom=0  CountResetPort=off  CountLoadPort=off  CountEnbPort=on  CountDirPort=off  CountHitOutputPort=off  CountDataType=Unsigned  CountWordLen=ceil(log2(hEnd))  CountFracLen=0  CountSampTime=1
  Logical Operator{3..6} (4 alike) : Logic  AllPortsSameDT=off  OutDataTypeStr=boolean
  Pixel Control Bus Creator : visionhdlutilities/Pixel Control Bus Creator
      settings: SourceProductBaseCode=VT
  Vertical : hdlsllib/Sources/HDL Counter  CountType=Count limited  CountInit=0  CountStep=1  CountMax=vEnd  CountFromType=Initial value  CountFrom=0  CountResetPort=off  CountLoadPort=off  CountEnbPort=on  CountDirPort=off  CountHitOutputPort=off  CountDataType=Unsigned  CountWordLen=ceil(log2(vEnd))  CountFracLen=0  CountSampTime=1
  hEnd : simulink/Logic and Bit Operations/Compare To Constant  relop===  const=hEnd  OutDataTypeStr=boolean
  hStart : simulink/Logic and Bit Operations/Compare To Constant  relop===  const=0  OutDataTypeStr=boolean
  vEnd : simulink/Logic and Bit Operations/Compare To Constant  relop===  const=vEnd  OutDataTypeStr=boolean
  vStart : simulink/Logic and Bit Operations/Compare To Constant  relop===  const=0  OutDataTypeStr=boolean
  busOut : Outport  VectorParamsAs1DForOutWhenUnconnected=off
  wires:
  validIn/1 -> Pixel Control Bus Creator/5, Vertical/1, Logical Operator4/1, Logical Operator5/1, Logical Operator6/1, Logical Operator3/1, Horizontal/1
  Horizontal/1 -> hEnd/1, hStart/1
  hEnd/1 -> Logical Operator4/2
  Vertical/1 -> vStart/1, vEnd/1
  vStart/1 -> Logical Operator5/2
  vEnd/1 -> Logical Operator6/2
  Logical Operator5/1 -> Pixel Control Bus Creator/3
  Logical Operator3/1 -> Pixel Control Bus Creator/1
  Logical Operator4/1 -> Pixel Control Bus Creator/2
  hStart/1 -> Logical Operator3/2
  Logical Operator6/1 -> Pixel Control Bus Creator/4
  Pixel Control Bus Creator/1 -> busOut/1

== system SGBMDisparityCopy/SGBMHDLAlgorithm/SGBMHDLAlgorithmWorker/MatchingCost/CensusTransform/validLogic/pixelBusGenerator ==
  validIn : Inport
  Horizontal : hdlsllib/Sources/HDL Counter  CountType=Count limited  CountInit=0  CountStep=1  CountMax=hEnd  CountFromType=Initial value  CountFrom=0  CountResetPort=off  CountLoadPort=off  CountEnbPort=on  CountDirPort=off  CountHitOutputPort=off  CountDataType=Unsigned  CountWordLen=ceil(log2(hEnd))  CountFracLen=0  CountSampTime=1
  Logical Operator{3..6} (4 alike) : Logic  AllPortsSameDT=off  OutDataTypeStr=boolean
  Pixel Control Bus Creator : visionhdlutilities/Pixel Control Bus Creator
      settings: SourceProductBaseCode=VT
  Vertical : hdlsllib/Sources/HDL Counter  CountType=Count limited  CountInit=0  CountStep=1  CountMax=vEnd  CountFromType=Initial value  CountFrom=0  CountResetPort=off  CountLoadPort=off  CountEnbPort=on  CountDirPort=off  CountHitOutputPort=off  CountDataType=Unsigned  CountWordLen=ceil(log2(vEnd))  CountFracLen=0  CountSampTime=1
  hEnd : simulink/Logic and Bit Operations/Compare To Constant  relop===  const=hEnd  OutDataTypeStr=boolean
  hStart : simulink/Logic and Bit Operations/Compare To Constant  relop===  const=0  OutDataTypeStr=boolean
  vEnd : simulink/Logic and Bit Operations/Compare To Constant  relop===  const=vEnd  OutDataTypeStr=boolean
  vStart : simulink/Logic and Bit Operations/Compare To Constant  relop===  const=0  OutDataTypeStr=boolean
  busOut : Outport  VectorParamsAs1DForOutWhenUnconnected=off
  wires:
  validIn/1 -> Pixel Control Bus Creator/5, Vertical/1, Logical Operator4/1, Logical Operator5/1, Logical Operator6/1, Logical Operator3/1, Horizontal/1
  Horizontal/1 -> hEnd/1, hStart/1
  hEnd/1 -> Logical Operator4/2
  Vertical/1 -> vStart/1, vEnd/1
  vStart/1 -> Logical Operator5/2
  vEnd/1 -> Logical Operator6/2
  Logical Operator5/1 -> Pixel Control Bus Creator/3
  Logical Operator3/1 -> Pixel Control Bus Creator/1
  Logical Operator4/1 -> Pixel Control Bus Creator/2
  hStart/1 -> Logical Operator3/2
  Logical Operator6/1 -> Pixel Control Bus Creator/4
  Pixel Control Bus Creator/1 -> busOut/1

== system SGBMDisparityCopy/SGBMHDLAlgorithm/SGBMHDLAlgorithmWorker/MatchingCost/CensusTransform/zeroPadding/FIFO ==
  dataIn : Inport
  Push : Inport  Port=2
  Pop : Inport  Port=3
  Reset : Inport  Port=4
  EmpltyFlag : RelationalOperator  Operator===  OutDataTypeStr=boolean  RndMeth=Nearest
  HDL Counter : hdlsllib/Sources/HDL Counter  CountType=Count limited  CountInit=0  CountStep=1  CountMax=((imgRowSize+6)*(imgColSize+8))-(imgRowSize*imgColSize)  CountFromType=Initial value  CountFrom=0  CountResetPort=on  CountLoadPort=off  CountEnbPort=on  CountDirPort=off  CountHitOutputPort=off  CountDataType=Unsigned  CountWordLen=ceil(log2(((imgRowSize+6)*(imgColSize+8))-(imgRowSize*imgColSize)))  CountFracLen=0  CountSampTime=1
  HDL Counter1 : hdlsllib/Sources/HDL Counter  CountType=Count limited  CountInit=0  CountStep=1  CountMax=((imgRowSize+6)*(imgColSize+8))-(imgRowSize*imgColSize)  CountFromType=Initial value  CountFrom=0  CountResetPort=on  CountLoadPort=off  CountEnbPort=on  CountDirPort=off  CountHitOutputPort=off  CountDataType=Unsigned  CountWordLen=ceil(log2(((imgRowSize+6)*(imgColSize+8))-(imgRowSize*imgColSize)))  CountFracLen=0  CountSampTime=1
  Simple Dual Port RAM : hdlsllib/HDL RAMs/Simple Dual Port RAM  ram_size=ceil(log2(((imgRowSize+6)*(imgColSize+8))-(imgRowSize*imgColSize)))
      settings: SourceProductBaseCode=SL
  dataOut : Outport  VectorParamsAs1DForOutWhenUnconnected=off
  empty : Outport  Port=2  VectorParamsAs1DForOutWhenUnconnected=off
  wires:
  HDL Counter1/1 -> EmpltyFlag/2, Simple Dual Port RAM/4
  Pop/1 -> HDL Counter1/2
  HDL Counter/1 -> EmpltyFlag/1, Simple Dual Port RAM/2
  Push/1 -> HDL Counter/2, Simple Dual Port RAM/3
  dataIn/1 -> Simple Dual Port RAM/1
  Simple Dual Port RAM/1 -> dataOut/1
  EmpltyFlag/1 -> empty/1
  Reset/1 -> HDL Counter1/1, HDL Counter/1

== system SGBMDisparityCopy/SGBMHDLAlgorithm/SGBMHDLAlgorithmWorker/MatchingCost/CensusTransform/zeroPadding/popSubsystem ==
  enable : Inport
  reset : Inport  Port=2
  Enable : EnablePort
  CC : simulink/Logic and Bit Operations/Compare To Constant  relop===  const=imgColSize+7  OutDataTypeStr=boolean
  CC1 : simulink/Logic and Bit Operations/Compare To Constant  relop=>=  const=3  OutDataTypeStr=boolean
  CC2 : simulink/Logic and Bit Operations/Compare To Constant  relop=>=  const=4  OutDataTypeStr=boolean
  CC3 : simulink/Logic and Bit Operations/Compare To Constant  relop=<  const=imgColSize+4  OutDataTypeStr=boolean
  CC4 : simulink/Logic and Bit Operations/Compare To Constant  relop=<  const=imgRowSize + 3  OutDataTypeStr=boolean
  CC6 : simulink/Logic and Bit Operations/Compare To Constant  relop===  const=imgRowSize + 5  OutDataTypeStr=boolean
  CC8 : simulink/Logic and Bit Operations/Compare To Constant  relop=>=  const=imgRowSize+2  OutDataTypeStr=boolean
  HDLC1 : hdlsllib/Sources/HDL Counter  CountType=Count limited  CountInit=0  CountStep=1  CountMax=imgColSize+7  CountFromType=Initial value  CountFrom=0  CountResetPort=on  CountLoadPort=off  CountEnbPort=on  CountDirPort=off  CountHitOutputPort=off  CountDataType=Unsigned  CountWordLen=ceil(log2(imgColSize+7))  CountFracLen=0  CountSampTime=1
  HDLC2 : hdlsllib/Sources/HDL Counter  CountType=Count limited  CountInit=0  CountStep=1  CountMax=imgRowSize+6  CountFromType=Initial value  CountFrom=0  CountResetPort=on  CountLoadPort=off  CountEnbPort=on  CountDirPort=off  CountHitOutputPort=off  CountDataType=Unsigned  CountWordLen=ceil(log2(imgRowSize+6))  CountFracLen=0  CountSampTime=1
  LO2 : Logic  Inputs=4  AllPortsSameDT=off  OutDataTypeStr=boolean
  LO4 : Logic  AllPortsSameDT=off  OutDataTypeStr=boolean
  done : Outport  InitialOutput=0  VectorParamsAs1DForOutWhenUnconnected=off
  pop : Outport  Port=2  InitialOutput=0  VectorParamsAs1DForOutWhenUnconnected=off
  lastRowOut : Outport  Port=3  InitialOutput=0  VectorParamsAs1DForOutWhenUnconnected=off
  wires:
  HDLC2/1 -> CC1/1, CC6/1, CC8/1, CC4/1
  CC4/1 -> LO2/2
  HDLC1/1 -> CC3/1, CC2/1, CC/1
  CC/1 -> HDLC2/2, LO4/1
  CC2/1 -> LO2/3
  CC3/1 -> LO2/4
  CC1/1 -> LO2/1
  CC6/1 -> LO4/2
  LO2/1 -> pop/1
  CC8/1 -> lastRowOut/1
  enable/1 -> HDLC1/2
  LO4/1 -> done/1
  reset/1 -> HDLC2/1, HDLC1/1

== system SGBMDisparityCopy/SGBMHDLAlgorithm/SGBMHDLAlgorithmWorker/MatchingCost/CensusTransform1/ctLogic/For Each Subsystem ==
  In1 : Inport  Partition=on  PartitionDimension=1  PartitionWidth=1  PartitionOffset=0
  In2 : Inport  Port=2  Partition=on  PartitionDimension=1  PartitionWidth=1  PartitionOffset=0
  For Each : ForEach  DisableCoverage=on
  Relational Operator : RelationalOperator  OutDataTypeStr=boolean  RndMeth=Nearest
  Out1 : Outport  ConcatenationDimension=1  VectorParamsAs1DForOutWhenUnconnected=off
  wires:
  In1/1 -> Relational Operator/1
  In2/1 -> Relational Operator/2
  Relational Operator/1 -> Out1/1

== system SGBMDisparityCopy/SGBMHDLAlgorithm/SGBMHDLAlgorithmWorker/MatchingCost/CensusTransform1/ctLogic/For Each Subsystem1 ==
  In1 : Inport  Partition=on  PartitionDimension=1  PartitionWidth=1  PartitionOffset=0
  In2 : Inport  Port=2  Partition=on  PartitionDimension=1  PartitionWidth=1  PartitionOffset=0
  For Each : ForEach  DisableCoverage=on
  Relational Operator : RelationalOperator  OutDataTypeStr=boolean  RndMeth=Nearest
  Out1 : Outport  ConcatenationDimension=1  VectorParamsAs1DForOutWhenUnconnected=off
  wires:
  In1/1 -> Relational Operator/1
  In2/1 -> Relational Operator/2
  Relational Operator/1 -> Out1/1

== system SGBMDisparityCopy/SGBMHDLAlgorithm/SGBMHDLAlgorithmWorker/MatchingCost/CensusTransform1/ctLogic/For Each Subsystem2 ==
  In1 : Inport  Partition=on  PartitionDimension=1  PartitionWidth=1  PartitionOffset=0
  In2 : Inport  Port=2  Partition=on  PartitionDimension=1  PartitionWidth=1  PartitionOffset=0
  For Each : ForEach  DisableCoverage=on
  Relational Operator : RelationalOperator  OutDataTypeStr=boolean  RndMeth=Nearest
  Out1 : Outport  ConcatenationDimension=1  VectorParamsAs1DForOutWhenUnconnected=off
  wires:
  In1/1 -> Relational Operator/1
  In2/1 -> Relational Operator/2
  Relational Operator/1 -> Out1/1

== system SGBMDisparityCopy/SGBMHDLAlgorithm/SGBMHDLAlgorithmWorker/MatchingCost/CensusTransform1/ctLogic/For Each Subsystem3 ==
  In1 : Inport  Partition=on  PartitionDimension=1  PartitionWidth=1  PartitionOffset=0
  In2 : Inport  Port=2  Partition=on  PartitionDimension=1  PartitionWidth=1  PartitionOffset=0
  For Each : ForEach  DisableCoverage=on
  Relational Operator : RelationalOperator  OutDataTypeStr=boolean  RndMeth=Nearest
  Out1 : Outport  ConcatenationDimension=1  VectorParamsAs1DForOutWhenUnconnected=off
  wires:
  In1/1 -> Relational Operator/1
  In2/1 -> Relational Operator/2
  Relational Operator/1 -> Out1/1

== system SGBMDisparityCopy/SGBMHDLAlgorithm/SGBMHDLAlgorithmWorker/MatchingCost/CensusTransform1/dataAligner/pixelBusGenerator ==
  validIn : Inport
  Horizontal : hdlsllib/Sources/HDL Counter  CountType=Count limited  CountInit=0  CountStep=1  CountMax=hEnd  CountFromType=Initial value  CountFrom=0  CountResetPort=off  CountLoadPort=off  CountEnbPort=on  CountDirPort=off  CountHitOutputPort=off  CountDataType=Unsigned  CountWordLen=ceil(log2(hEnd))  CountFracLen=0  CountSampTime=1
  Logical Operator{3..6} (4 alike) : Logic  AllPortsSameDT=off  OutDataTypeStr=boolean
  Pixel Control Bus Creator : visionhdlutilities/Pixel Control Bus Creator
      settings: SourceProductBaseCode=VT
  Vertical : hdlsllib/Sources/HDL Counter  CountType=Count limited  CountInit=0  CountStep=1  CountMax=vEnd  CountFromType=Initial value  CountFrom=0  CountResetPort=off  CountLoadPort=off  CountEnbPort=on  CountDirPort=off  CountHitOutputPort=off  CountDataType=Unsigned  CountWordLen=ceil(log2(vEnd))  CountFracLen=0  CountSampTime=1
  hEnd : simulink/Logic and Bit Operations/Compare To Constant  relop===  const=hEnd  OutDataTypeStr=boolean
  hStart : simulink/Logic and Bit Operations/Compare To Constant  relop===  const=0  OutDataTypeStr=boolean
  vEnd : simulink/Logic and Bit Operations/Compare To Constant  relop===  const=vEnd  OutDataTypeStr=boolean
  vStart : simulink/Logic and Bit Operations/Compare To Constant  relop===  const=0  OutDataTypeStr=boolean
  busOut : Outport  VectorParamsAs1DForOutWhenUnconnected=off
  wires:
  validIn/1 -> Pixel Control Bus Creator/5, Vertical/1, Logical Operator4/1, Logical Operator5/1, Logical Operator6/1, Logical Operator3/1, Horizontal/1
  Horizontal/1 -> hEnd/1, hStart/1
  hEnd/1 -> Logical Operator4/2
  Vertical/1 -> vStart/1, vEnd/1
  vStart/1 -> Logical Operator5/2
  vEnd/1 -> Logical Operator6/2
  Logical Operator5/1 -> Pixel Control Bus Creator/3
  Logical Operator3/1 -> Pixel Control Bus Creator/1
  Logical Operator4/1 -> Pixel Control Bus Creator/2
  hStart/1 -> Logical Operator3/2
  Logical Operator6/1 -> Pixel Control Bus Creator/4
  Pixel Control Bus Creator/1 -> busOut/1
